simulink model "VTOLAutopilotController (minhyun-purdue's conflicted copy 2025-07-07)"  (R2024b)
settings: configuration reference "VTOLConfiguration" (kept outside this file)
undefined symbols (not defined in the file): control, controlParams, ControlSampleTime, CriticalTiltAngle, DiscIntNeverNeededParam, dspblkCoreblockFVToolHelper, flightState, FSState, FWControlParams, FWTrimSpeed, gcbh, HoverMission, R_LOOKAHEAD, ReferenceFilterDen, ReferenceFilterNum, tilt_max, tiltIni, uavParam, VTOLcontrolGains, w_trim, WindDownRate
libraries: slpidlib x32, simulink x11, uavalgslib x7, simulink_extras x1
(part 3 of 6)

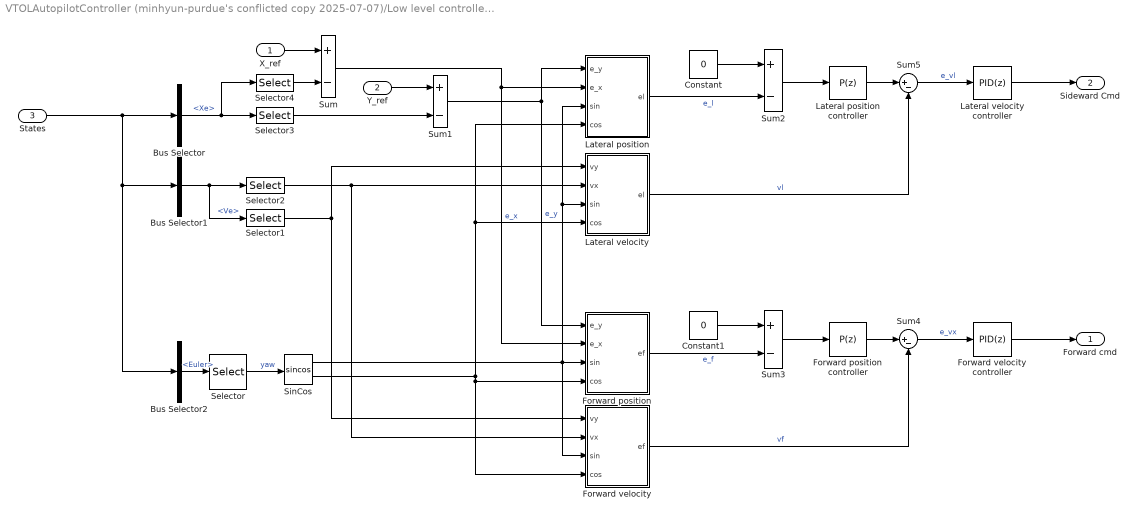
== system VTOLAutopilotController (minhyun-purdue's conflicted copy 2025-07-07)/Low level controller/Multicopter Controller/Horizontal Position Control/XY Controller ==
  X_ref : Inport
  Y_ref : Inport  Port=2
  States : Inport  Port=3
  Bus Selector : BusSelector  OutputSignals=Xe
  Bus Selector1 : BusSelector  OutputSignals=Ve
  Bus Selector2 : BusSelector  OutputSignals=Euler
  Constant : Constant  Value=0
  Constant1 : Constant  Value=0
  Forward position : Subsystem
  Forward position controller : slpidlib/PID Controller  Controller=P  Form=Parallel  TimeDomain=Discrete-time  UseExternalTs=off  SampleTime=-1  IntegratorMethod=Forward Euler  FilterMethod=Forward Euler  ControllerParametersSource=internal  P=VTOLcontrolGains.P_X  I=controlParams.I_X  UseKiTs=off  D=0.741088334151374  UseExternalDerivativeSource=off  N=1.14081860742283  UseFilter=on  TunerSelectOption=Transfer Function Based (PID Tuner App)  InitialConditionSource=internal  InitialConditionForIntegrator=0  InitialConditionForFilter=0  DifferentiatorICPrevScaledInput=0  ExternalReset=none  TrackingMode=off  Kt=1  LimitOutput=off  SatLimitsSource=internal  UpperSaturationLimit=inf  LowerSaturationLimit=-inf  LinearizeAsGain=on  AntiWindupMode=none  Kb=1  LimitIntegrator=off  UpperIntegratorSaturationLimit=inf  LowerIntegratorSaturationLimit=-inf  POutMin=[]  POutMax=[]  IOutMin=[]  IOutMax=[]  DOutMin=[]  DOutMax=[]  NOutMin=[]  NOutMax=[]  SumOutMin=[]  SumOutMax=[]  SaturationOutMin=[]  SaturationOutMax=[]  PParamMin=[]  PParamMax=[]  IParamMin=[]  IParamMax=[]  DParamMin=[]  DParamMax=[]  NParamMin=[]  NParamMax=[]  KbParamMin=[]  KbParamMax=[]  KtParamMin=[]  KtParamMax=[]  KbOutMin=[]  KbOutMax=[]  KtOutMin=[]  KtOutMax=[]  IntegratorOutMin=[]  IntegratorOutMax=[]  FilterOutMin=[]  FilterOutMax=[]  SumI1OutMin=[]  SumI1OutMax=[]  SumI2OutMin=[]  SumI2OutMax=[]  SumI3OutMin=[]  SumI3OutMax=[]  SumI4OutMin=[]  SumI4OutMax=[]  SumDOutMin=[]  SumDOutMax=[]  DifferentiatorOutMin=[]  DifferentiatorOutMax=[]  FilterDiffOutCoefMin=[]  FilterDiffOutCoefMax=[]  ReciprocalOutMin=[]  ReciprocalOutMax=[]  SumDenOutMin=[]  SumDenOutMax=[]  SumNumOutMin=[]  SumNumOutMax=[]  DivideOutMin=[]  DivideOutMax=[]  UdiffTsProdOutMin=[]  UdiffTsProdOutMax=[]  NTsProdOutMin=[]  NTsProdOutMax=[]  UintegralTsProdOutMin=[]  UintegralTsProdOutMax=[]  UngainTsProdOutMin=[]  UngainTsProdOutMax=[]  ClampingZeroOutDataTypeStr=Inherit: Inherit via back propagation  ClampingZeroOutMin=[]  ClampingZeroOutMax=[]  FilterDenConstantOutDataTypeStr=Inherit: Inherit via back propagation  FilterDenConstantOutMin=[]  FilterDenConstantOutMax=[]  PCopyOutDataTypeStr=Inherit: Inherit via back propagation  PCopyOutMin=[]  PCopyOutMax=[]  NCopyOutDataTypeStr=Inherit: Inherit via back propagation  NCopyOutMin=[]  NCopyOutMax=[]  IntegratorContinuousStateAttributes=''  IntegratorStateMustResolveToSignalObject=off  IntegratorRTWStateStorageClass=Auto  FilterContinuousStateAttributes=''  FilterStateMustResolveToSignalObject=off  FilterRTWStateStorageClass=Auto  ParallelPVariant=InternalParameters  IdealPVariant=Disabled  IVariant=Disabled  DVariant=Disabled  IntegratorVariant=Disabled  SatVariant=Disabled  AWVariant=Disabled  PCopyVariant=Disabled  TRVariant=Disabled  FdbkBlocksVariant=Forward  IdealPFdbkVariant=Disabled  SatFdbkVariant=Disabled  DerivativeFilterVariant=Disabled  NVariant=Disabled  NCopyVariant=Disabled_SignalSpec  FilterICVariant=Disabled  IntegratorICVariant=Disabled  ExternalResetVariant=Disabled  TRSumVariant=Passthrough  SumFdbkVariant=Disabled  SumVariant=Passthrough_P  TsampFilterVariant=InternalTs  TsampNgainVariant=Passthrough  TsampIntegralVariant=Disabled_SignalSpec  ExternalSaturationOutDataTypeStr=Inherit: Same as second input  DerivativeSourceVariant=Disabled  PreIntVariant=InternalPreInt
  Forward velocity : Subsystem
  Forward velocity controller : slpidlib/PID Controller  Controller=PID  Form=Parallel  TimeDomain=Discrete-time  UseExternalTs=off  SampleTime=-1  IntegratorMethod=Forward Euler  FilterMethod=Forward Euler  ControllerParametersSource=internal  P=VTOLcontrolGains.P_VX  I=VTOLcontrolGains.I_VX  UseKiTs=off  D=VTOLcontrolGains.D_VX  UseExternalDerivativeSource=off  N=VTOLcontrolGains.N_VX  UseFilter=on  TunerSelectOption=Transfer Function Based (PID Tuner App)  InitialConditionSource=internal  InitialConditionForIntegrator=0  InitialConditionForFilter=0  DifferentiatorICPrevScaledInput=0  ExternalReset=none  TrackingMode=off  Kt=1  LimitOutput=off  SatLimitsSource=internal  UpperSaturationLimit=inf  LowerSaturationLimit=-inf  LinearizeAsGain=on  AntiWindupMode=none  Kb=1  LimitIntegrator=off  UpperIntegratorSaturationLimit=inf  LowerIntegratorSaturationLimit=-inf  POutMin=[]  POutMax=[]  IOutMin=[]  IOutMax=[]  DOutMin=[]  DOutMax=[]  NOutMin=[]  NOutMax=[]  SumOutMin=[]  SumOutMax=[]  SaturationOutMin=[]  SaturationOutMax=[]  PParamMin=[]  PParamMax=[]  IParamMin=[]  IParamMax=[]  DParamMin=[]  DParamMax=[]  NParamMin=[]  NParamMax=[]  KbParamMin=[]  KbParamMax=[]  KtParamMin=[]  KtParamMax=[]  KbOutMin=[]  KbOutMax=[]  KtOutMin=[]  KtOutMax=[]  IntegratorOutMin=[]  IntegratorOutMax=[]  FilterOutMin=[]  FilterOutMax=[]  SumI1OutMin=[]  SumI1OutMax=[]  SumI2OutMin=[]  SumI2OutMax=[]  SumI3OutMin=[]  SumI3OutMax=[]  SumI4OutMin=[]  SumI4OutMax=[]  SumDOutMin=[]  SumDOutMax=[]  DifferentiatorOutMin=[]  DifferentiatorOutMax=[]  FilterDiffOutCoefMin=[]  FilterDiffOutCoefMax=[]  ReciprocalOutMin=[]  ReciprocalOutMax=[]  SumDenOutMin=[]  SumDenOutMax=[]  SumNumOutMin=[]  SumNumOutMax=[]  DivideOutMin=[]  DivideOutMax=[]  UdiffTsProdOutMin=[]  UdiffTsProdOutMax=[]  NTsProdOutMin=[]  NTsProdOutMax=[]  UintegralTsProdOutMin=[]  UintegralTsProdOutMax=[]  UngainTsProdOutMin=[]  UngainTsProdOutMax=[]  ClampingZeroOutDataTypeStr=Inherit: Inherit via back propagation  ClampingZeroOutMin=[]  ClampingZeroOutMax=[]  FilterDenConstantOutDataTypeStr=Inherit: Inherit via back propagation  FilterDenConstantOutMin=[]  FilterDenConstantOutMax=[]  PCopyOutDataTypeStr=Inherit: Inherit via back propagation  PCopyOutMin=[]  PCopyOutMax=[]  NCopyOutDataTypeStr=Inherit: Inherit via back propagation  NCopyOutMin=[]  NCopyOutMax=[]  IntegratorContinuousStateAttributes=''  IntegratorStateMustResolveToSignalObject=off  IntegratorRTWStateStorageClass=Auto  FilterContinuousStateAttributes=''  FilterStateMustResolveToSignalObject=off  FilterRTWStateStorageClass=Auto  ParallelPVariant=InternalParameters  IdealPVariant=Disabled  IVariant=InternalParameters  DVariant=InternalParameters  IntegratorVariant=Discrete  SatVariant=Disabled  AWVariant=Passthrough  PCopyVariant=Disabled  TRVariant=Disabled  FdbkBlocksVariant=Forward  IdealPFdbkVariant=Disabled  SatFdbkVariant=Disabled  DerivativeFilterVariant=ForwardEulerFilter  NVariant=InternalParameters  NCopyVariant=Disabled  FilterICVariant=InternalICsFilter  IntegratorICVariant=InternalICs  ExternalResetVariant=Disabled  TRSumVariant=Passthrough  SumFdbkVariant=Disabled  SumVariant=Sum_PID  TsampFilterVariant=InternalTs  TsampNgainVariant=Passthrough  TsampIntegralVariant=Disabled_SignalSpec  ExternalSaturationOutDataTypeStr=Inherit: Same as second input  DerivativeSourceVariant=ErrorSignal  PreIntVariant=InternalPreInt
  Lateral position : Subsystem
  Lateral position controller : slpidlib/PID Controller  Controller=P  Form=Parallel  TimeDomain=Discrete-time  UseExternalTs=off  SampleTime=-1  IntegratorMethod=Forward Euler  FilterMethod=Forward Euler  ControllerParametersSource=internal  P=VTOLcontrolGains.P_Y  I=controlParams.I_Y  UseKiTs=off  D=0.20966837124708  UseExternalDerivativeSource=off  N=1.18305565097938  UseFilter=on  TunerSelectOption=Transfer Function Based (PID Tuner App)  InitialConditionSource=internal  InitialConditionForIntegrator=0  InitialConditionForFilter=0  DifferentiatorICPrevScaledInput=0  ExternalReset=none  TrackingMode=off  Kt=1  LimitOutput=off  SatLimitsSource=internal  UpperSaturationLimit=0.4  LowerSaturationLimit=-0.4  LinearizeAsGain=on  AntiWindupMode=clamping  Kb=1  LimitIntegrator=off  UpperIntegratorSaturationLimit=inf  LowerIntegratorSaturationLimit=-inf  POutMin=[]  POutMax=[]  IOutMin=[]  IOutMax=[]  DOutMin=[]  DOutMax=[]  NOutMin=[]  NOutMax=[]  SumOutMin=[]  SumOutMax=[]  SaturationOutMin=[]  SaturationOutMax=[]  PParamMin=[]  PParamMax=[]  IParamMin=[]  IParamMax=[]  DParamMin=[]  DParamMax=[]  NParamMin=[]  NParamMax=[]  KbParamMin=[]  KbParamMax=[]  KtParamMin=[]  KtParamMax=[]  KbOutMin=[]  KbOutMax=[]  KtOutMin=[]  KtOutMax=[]  IntegratorOutMin=[]  IntegratorOutMax=[]  FilterOutMin=[]  FilterOutMax=[]  SumI1OutMin=[]  SumI1OutMax=[]  SumI2OutMin=[]  SumI2OutMax=[]  SumI3OutMin=[]  SumI3OutMax=[]  SumI4OutMin=[]  SumI4OutMax=[]  SumDOutMin=[]  SumDOutMax=[]  DifferentiatorOutMin=[]  DifferentiatorOutMax=[]  FilterDiffOutCoefMin=[]  FilterDiffOutCoefMax=[]  ReciprocalOutMin=[]  ReciprocalOutMax=[]  SumDenOutMin=[]  SumDenOutMax=[]  SumNumOutMin=[]  SumNumOutMax=[]  DivideOutMin=[]  DivideOutMax=[]  UdiffTsProdOutMin=[]  UdiffTsProdOutMax=[]  NTsProdOutMin=[]  NTsProdOutMax=[]  UintegralTsProdOutMin=[]  UintegralTsProdOutMax=[]  UngainTsProdOutMin=[]  UngainTsProdOutMax=[]  ClampingZeroOutDataTypeStr=Inherit: Inherit via back propagation  ClampingZeroOutMin=[]  ClampingZeroOutMax=[]  FilterDenConstantOutDataTypeStr=Inherit: Inherit via back propagation  FilterDenConstantOutMin=[]  FilterDenConstantOutMax=[]  PCopyOutDataTypeStr=Inherit: Inherit via back propagation  PCopyOutMin=[]  PCopyOutMax=[]  NCopyOutDataTypeStr=Inherit: Inherit via back propagation  NCopyOutMin=[]  NCopyOutMax=[]  IntegratorContinuousStateAttributes=''  IntegratorStateMustResolveToSignalObject=off  IntegratorRTWStateStorageClass=Auto  FilterContinuousStateAttributes=''  FilterStateMustResolveToSignalObject=off  FilterRTWStateStorageClass=Auto  ParallelPVariant=InternalParameters  IdealPVariant=Disabled  IVariant=Disabled  DVariant=Disabled  IntegratorVariant=Disabled  SatVariant=Disabled  AWVariant=Disabled  PCopyVariant=Disabled  TRVariant=Disabled  FdbkBlocksVariant=Forward  IdealPFdbkVariant=Disabled  SatFdbkVariant=Disabled  DerivativeFilterVariant=Disabled  NVariant=Disabled  NCopyVariant=Disabled_SignalSpec  FilterICVariant=Disabled  IntegratorICVariant=Disabled  ExternalResetVariant=Disabled  TRSumVariant=Passthrough  SumFdbkVariant=Disabled  SumVariant=Passthrough_P  TsampFilterVariant=InternalTs  TsampNgainVariant=Passthrough  TsampIntegralVariant=Disabled_SignalSpec  ExternalSaturationOutDataTypeStr=Inherit: Same as second input  DerivativeSourceVariant=Disabled  PreIntVariant=InternalPreInt
  Lateral velocity : Subsystem
  "Lateral velocity controller " : slpidlib/PID Controller  Controller=PID  Form=Parallel  TimeDomain=Discrete-time  UseExternalTs=off  SampleTime=-1  IntegratorMethod=Forward Euler  FilterMethod=Forward Euler  ControllerParametersSource=internal  P=VTOLcontrolGains.P_VY  I=VTOLcontrolGains.I_VY  UseKiTs=off  D=VTOLcontrolGains.D_VY  UseExternalDerivativeSource=off  N=VTOLcontrolGains.N_VY  UseFilter=on  TunerSelectOption=Transfer Function Based (PID Tuner App)  InitialConditionSource=internal  InitialConditionForIntegrator=0  InitialConditionForFilter=0  DifferentiatorICPrevScaledInput=0  ExternalReset=none  TrackingMode=off  Kt=1  LimitOutput=off  SatLimitsSource=internal  UpperSaturationLimit=inf  LowerSaturationLimit=-inf  LinearizeAsGain=on  AntiWindupMode=none  Kb=1  LimitIntegrator=off  UpperIntegratorSaturationLimit=inf  LowerIntegratorSaturationLimit=-inf  POutMin=[]  POutMax=[]  IOutMin=[]  IOutMax=[]  DOutMin=[]  DOutMax=[]  NOutMin=[]  NOutMax=[]  SumOutMin=[]  SumOutMax=[]  SaturationOutMin=[]  SaturationOutMax=[]  PParamMin=[]  PParamMax=[]  IParamMin=[]  IParamMax=[]  DParamMin=[]  DParamMax=[]  NParamMin=[]  NParamMax=[]  KbParamMin=[]  KbParamMax=[]  KtParamMin=[]  KtParamMax=[]  KbOutMin=[]  KbOutMax=[]  KtOutMin=[]  KtOutMax=[]  IntegratorOutMin=[]  IntegratorOutMax=[]  FilterOutMin=[]  FilterOutMax=[]  SumI1OutMin=[]  SumI1OutMax=[]  SumI2OutMin=[]  SumI2OutMax=[]  SumI3OutMin=[]  SumI3OutMax=[]  SumI4OutMin=[]  SumI4OutMax=[]  SumDOutMin=[]  SumDOutMax=[]  DifferentiatorOutMin=[]  DifferentiatorOutMax=[]  FilterDiffOutCoefMin=[]  FilterDiffOutCoefMax=[]  ReciprocalOutMin=[]  ReciprocalOutMax=[]  SumDenOutMin=[]  SumDenOutMax=[]  SumNumOutMin=[]  SumNumOutMax=[]  DivideOutMin=[]  DivideOutMax=[]  UdiffTsProdOutMin=[]  UdiffTsProdOutMax=[]  NTsProdOutMin=[]  NTsProdOutMax=[]  UintegralTsProdOutMin=[]  UintegralTsProdOutMax=[]  UngainTsProdOutMin=[]  UngainTsProdOutMax=[]  ClampingZeroOutDataTypeStr=Inherit: Inherit via back propagation  ClampingZeroOutMin=[]  ClampingZeroOutMax=[]  FilterDenConstantOutDataTypeStr=Inherit: Inherit via back propagation  FilterDenConstantOutMin=[]  FilterDenConstantOutMax=[]  PCopyOutDataTypeStr=Inherit: Inherit via back propagation  PCopyOutMin=[]  PCopyOutMax=[]  NCopyOutDataTypeStr=Inherit: Inherit via back propagation  NCopyOutMin=[]  NCopyOutMax=[]  IntegratorContinuousStateAttributes=''  IntegratorStateMustResolveToSignalObject=off  IntegratorRTWStateStorageClass=Auto  FilterContinuousStateAttributes=''  FilterStateMustResolveToSignalObject=off  FilterRTWStateStorageClass=Auto  ParallelPVariant=InternalParameters  IdealPVariant=Disabled  IVariant=InternalParameters  DVariant=InternalParameters  IntegratorVariant=Discrete  SatVariant=Disabled  AWVariant=Passthrough  PCopyVariant=Disabled  TRVariant=Disabled  FdbkBlocksVariant=Forward  IdealPFdbkVariant=Disabled  SatFdbkVariant=Disabled  DerivativeFilterVariant=ForwardEulerFilter  NVariant=InternalParameters  NCopyVariant=Disabled  FilterICVariant=InternalICsFilter  IntegratorICVariant=InternalICs  ExternalResetVariant=Disabled  TRSumVariant=Passthrough  SumFdbkVariant=Disabled  SumVariant=Sum_PID  TsampFilterVariant=InternalTs  TsampNgainVariant=Passthrough  TsampIntegralVariant=Disabled_SignalSpec  ExternalSaturationOutDataTypeStr=Inherit: Same as second input  DerivativeSourceVariant=ErrorSignal  PreIntVariant=InternalPreInt
  Selector : Selector  InputPortWidth=3  IndexOptions=Index vector (dialog)  Indices=[3]  OutputSizes=1
  Selector1 : Selector  InputPortWidth=3  IndexOptions=Index vector (dialog)  Indices=[2]  OutputSizes=1
  Selector2 : Selector  InputPortWidth=3  IndexOptions=Index vector (dialog)  Indices=[1]  OutputSizes=1
  Selector3 : Selector  InputPortWidth=3  IndexOptions=Index vector (dialog)  Indices=[2]  OutputSizes=1
  Selector4 : Selector  InputPortWidth=3  IndexOptions=Index vector (dialog)  Indices=[1]  OutputSizes=1
  SinCos : Trigonometry  Operator=sincos
  Sum{,1..3} (4 alike) : Sum  Inputs=+-
  Sum4 : Sum  Inputs=|+-
  Sum5 : Sum  Inputs=|+-
  Forward cmd : Outport
  Sideward Cmd : Outport  Port=2
  wires:
  States/1 -> Bus Selector2/1, Bus Selector1/1, Bus Selector/1
  Bus Selector/1 -> Selector4/1, Selector3/1  "<Xe>"
  Y_ref/1 -> Sum1/1
  Sum4/1 -> Forward velocity controller/1  "e_vx"
  SinCos/2 -> Forward velocity/4(cos), Forward position/4(cos), Lateral position/4(cos), Lateral velocity/4(cos)
  Selector/1 -> SinCos/1  "yaw"
  Lateral position/1(el) -> Sum2/2  "e_l"
  Sum1/1 -> Lateral position/1(e_y), Forward position/1(e_y)  "e_y"
  SinCos/1 -> Lateral velocity/3(sin), Lateral position/3(sin), Forward position/3(sin), Forward velocity/3(sin)
  Lateral velocity/1(el) -> Sum5/2  "vl"
  Forward position/1(ef) -> Sum3/2  "e_f"
  Forward velocity/1(ef) -> Sum4/2  "vf"
  Lateral position controller/1 -> Sum5/1
  Forward position controller/1 -> Sum4/1
  Sum5/1 -> "Lateral velocity controller "/1  "e_vl"
  "Lateral velocity controller "/1 -> Sideward Cmd/1
  Forward velocity controller/1 -> Forward cmd/1
  Constant/1 -> Sum2/1
  Sum2/1 -> Lateral position controller/1
  Constant1/1 -> Sum3/1
  Sum3/1 -> Forward position controller/1
  Bus Selector2/1 -> Selector/1  "<Euler>"
  Selector2/1 -> Forward velocity/2(vx), Lateral velocity/2(vx)
  Selector1/1 -> Lateral velocity/1(vy), Forward velocity/1(vy)
  Bus Selector1/1 -> Selector2/1, Selector1/1  "<Ve>"
  Selector3/1 -> Sum1/2
  Selector4/1 -> Sum/2
  Sum/1 -> Forward position/2(e_x), Lateral position/2(e_x)  "e_x"
  X_ref/1 -> Sum/1

== system VTOLAutopilotController (minhyun-purdue's conflicted copy 2025-07-07)/Low level controller/Multicopter Controller/Subsystem/Triggered Subsystem ==
  YawHold : Inport
  Trigger : TriggerPort  VariantControl=(inherit)
  Reference : Outport
  wires:
  YawHold/1 -> Reference/1

== system VTOLAutopilotController (minhyun-purdue's conflicted copy 2025-07-07)/Low level controller/Scheduler/FixedWingScheduler/Switch Case Action Subsystem ==
  note: No control allocated from fixed wing during hover.
  Action Port : ActionPort  ActionPortLabel=case [ Hover ]:
  Bus Creator : BusCreator  Inputs=4
  Constant{,1..3} (4 alike) : Constant  Value=0
  FixedWingControls : Outport  OutDataTypeStr=Bus: FixedWingCtrlBus
  wires:
  Bus Creator/1 -> FixedWingControls/1
  Constant/1 -> Bus Creator/1  "dA"
  Constant1/1 -> Bus Creator/2  "dE"
  Constant2/1 -> Bus Creator/3  "dR"
  Constant3/1 -> Bus Creator/4  "dT"

== system VTOLAutopilotController (minhyun-purdue's conflicted copy 2025-07-07)/Low level controller/Scheduler/FixedWingScheduler/Switch Case Action Subsystem1 ==
  FixedWingActuators : Inport  OutDataTypeStr=Bus: FixedWingCtrlBus
  TransitionDone : Inport  Port=2
  Action Port : ActionPort  ActionPortLabel=case [ Transition ]:
  Bus Creator : BusCreator  Inputs=4  OutDataTypeStr=Bus: FixedWingCtrlBus
  Constant : Constant  Value=0
  Constant1 : Constant  Value=controlParams.FWElevatorTrim
  Constant2 : Constant  Value=0
  Constant3 : Constant  Value=0
  Switch : Switch  Criteria=u2 > Threshold  SaturateOnIntegerOverflow=off  InputSameDT=off
  FixedWingControls : Outport  OutDataTypeStr=Bus: FixedWingCtrlBus
  wires:
  Bus Creator/1 -> Switch/3
  Constant/1 -> Bus Creator/1  "dA"
  Constant1/1 -> Bus Creator/2  "dE"
  Constant2/1 -> Bus Creator/3  "dR"
  Constant3/1 -> Bus Creator/4  "dT"
  FixedWingActuators/1 -> Switch/1
  Switch/1 -> FixedWingControls/1
  TransitionDone/1 -> Switch/2

== system VTOLAutopilotController (minhyun-purdue's conflicted copy 2025-07-07)/Low level controller/Scheduler/FixedWingScheduler/Switch Case Action Subsystem2 ==
  FixedWingActuators : Inport  OutDataTypeStr=Bus: FixedWingCtrlBus
  Action Port : ActionPort  ActionPortLabel=case [ FixedWing ]:
  FixedWingControls : Outport  OutDataTypeStr=Bus: FixedWingCtrlBus
  wires:
  FixedWingActuators/1 -> FixedWingControls/1

== system VTOLAutopilotController (minhyun-purdue's conflicted copy 2025-07-07)/Low level controller/Scheduler/FixedWingScheduler/Switch Case Action Subsystem3 ==
  note: No control allocated from fixed wing during hover.
  Action Port : ActionPort  ActionPortLabel=case [ BackTransition ]:
  Bus Creator : BusCreator  Inputs=4
  Constant{,1..3} (4 alike) : Constant  Value=0
  FixedWingControls : Outport  OutDataTypeStr=Bus: FixedWingCtrlBus
  wires:
  Bus Creator/1 -> FixedWingControls/1
  Constant/1 -> Bus Creator/1  "dA"
  Constant1/1 -> Bus Creator/2  "dE"
  Constant3/1 -> Bus Creator/4  "dT"
  Constant2/1 -> Bus Creator/3  "dR"

== system VTOLAutopilotController (minhyun-purdue's conflicted copy 2025-07-07)/Low level controller/Scheduler/Subsystem/Actuator To Voltage ==
  note: #2, 25/05/20, MH, Fixed
      | The rotor rotational speed command should be
      | normalized to [rad/s].Previously, division by 2PI
      | was omitted in the command block,
      | while the 'Rotor Assembly' block multiplies
      | the input by 2PI, leading to increased gains.
  Motor Commands : Inport
  Bus Creator : BusCreator  Inputs=6  OutDataTypeStr=Bus: RotorCtrlBus
  Bus Selector : BusSelector  OutputSignals=w1,w2,w3,w4,Tilt1,Tilt2
  Gain{,1..2,4} (4 alike) : Gain  Gain=1/(uavParam.motor.RPMMAX/60)
  Gain3 : Gain  Gain=1/(pi/2)
  Gain5 : Gain  Gain=1/(pi/2)
  Gain{6..9} (4 alike) : Gain  Gain=1/(2*pi)
  Saturation{,1..3} (4 alike) : Saturate  UpperLimit=controlParams.maxPWM  LowerLimit=controlParams.minPWM
  Saturation4 : Saturate  UpperLimit=1  LowerLimit=0
  Saturation5 : Saturate  UpperLimit=1  LowerLimit=0
  To PWM : Outport
  wires:
  Motor Commands/1 -> Bus Selector/1
  Bus Selector/1 -> Gain/1  "<w1>"
  Bus Selector/3 -> Gain1/1  "<w3>"
  Bus Selector/2 -> Gain4/1  "<w2>"
  Bus Selector/4 -> Gain2/1  "<w4>"
  Bus Selector/5 -> Gain3/1  "<Tilt1>"
  Bus Selector/6 -> Gain5/1  "<Tilt2>"
  Gain/1 -> Gain6/1  "w1"
  Gain4/1 -> Gain7/1  "w2"
  Gain1/1 -> Gain8/1  "w3"
  Gain2/1 -> Gain9/1  "w4"
  Gain3/1 -> Saturation4/1
  Gain5/1 -> Saturation5/1
  Bus Creator/1 -> To PWM/1
  Gain6/1 -> Saturation/1
  Gain7/1 -> Saturation1/1
  Gain8/1 -> Saturation2/1
  Gain9/1 -> Saturation3/1
  Saturation/1 -> Bus Creator/1  "w1"
  Saturation1/1 -> Bus Creator/2  "w2"
  Saturation2/1 -> Bus Creator/3  "w3"
  Saturation3/1 -> Bus Creator/4  "w4"
  Saturation4/1 -> Bus Creator/5  "Tilt1"
  Saturation5/1 -> Bus Creator/6  "Tilt2"

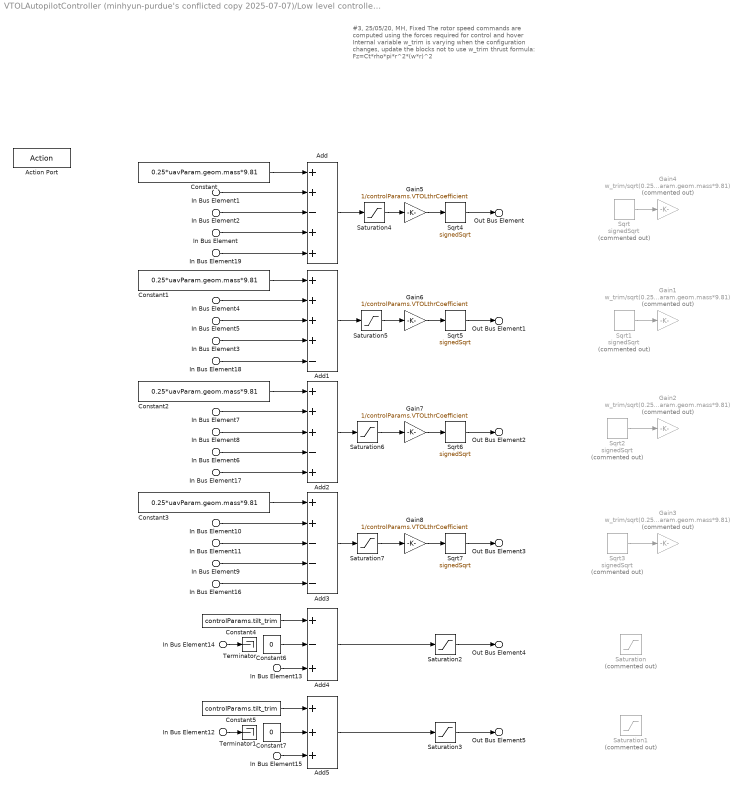
== system VTOLAutopilotController (minhyun-purdue's conflicted copy 2025-07-07)/Low level controller/Scheduler/Subsystem/Switch Case Action Subsystem ==
  note: #3, 25/05/20, MH, Fixed
      | The rotor speed commands are computed using
      | the forces required for control and hover
      | Internal variable w_trim is varying when the
      | configuration changes, update the blocks not to
      | use w_trim
      | thrust formula: Fz=Ct*rho*pi*r^2*(w*r)^2
  In Bus Element{,3,6,9} (4 alike) : Inport  PortName=MixerCommands  Element=w_theta
  In Bus Element{1,4,7,10} (4 alike) : Inport  PortName=MixerCommands  Element=w_z
  In Bus Element{2,5,8,11} (4 alike) : Inport  PortName=MixerCommands  Element=w_phi
  In Bus Element13 : Inport  PortName=MixerCommands  Element=l_x
  In Bus Element15 : Inport  PortName=MixerCommands  Element=l_x
  In Bus Element{12,14,16..19} (6 alike) : Inport  PortName=MixerCommands  Element=w_psi
  Action Port : ActionPort  ActionPortLabel=case [ Hover ]:
  Add : Sum  Inputs=++-++
  Add1 : Sum  Inputs=++++-
  Add2 : Sum  Inputs=+++-+
  Add3 : Sum  Inputs=++---
  Add4 : Sum  Inputs=+-+
  Add5 : Sum  Inputs=+++
  Constant{,1..3} (4 alike) : Constant  Value=0.25*uavParam.geom.mass*9.81
  Constant4 : Constant  Value=controlParams.tilt_trim
  Constant5 : Constant  Value=controlParams.tilt_trim
  Constant6 : Constant  Value=0
  Constant7 : Constant  Value=0
  Gain{1..4} (4 alike) : Gain  Commented=on  Gain=w_trim/sqrt(0.25*uavParam.geom.mass*9.81)
  Gain{5..8} (4 alike) : Gain  Gain=1/controlParams.VTOLthrCoefficient
  Saturation : Saturate  Commented=on  UpperLimit=tilt_max  LowerLimit=-tilt_max
  Saturation1 : Saturate  Commented=on  UpperLimit=tilt_max  LowerLimit=-tilt_max
  Saturation2 : Saturate  UpperLimit=tilt_max  LowerLimit=-tilt_max
  Saturation3 : Saturate  UpperLimit=tilt_max  LowerLimit=-tilt_max
  Saturation{4..7} (4 alike) : Saturate  UpperLimit=inf  LowerLimit=0
  Sqrt{,1..3} (4 alike) : Sqrt  Commented=on  Operator=signedSqrt
  Sqrt{4..7} (4 alike) : Sqrt  Operator=signedSqrt
  Terminator : Terminator
  Terminator1 : Terminator
  Out Bus Element : Outport  PortName=Actuator  Element=w1
  Out Bus Element1 : Outport  PortName=Actuator  Element=w2
  Out Bus Element2 : Outport  PortName=Actuator  Element=w3
  Out Bus Element3 : Outport  PortName=Actuator  Element=w4
  Out Bus Element4 : Outport  PortName=Actuator  Element=Tilt1
  Out Bus Element5 : Outport  PortName=Actuator  Element=Tilt2
  wires:
  Constant5/1 -> Add5/1
  Constant2/1 -> Add2/1
  Constant1/1 -> Add1/1
  Constant4/1 -> Add4/1
  Constant/1 -> Add/1
  Constant3/1 -> Add3/1
  Add/1 -> Saturation4/1
  Add1/1 -> Saturation5/1
  Add2/1 -> Saturation6/1
  Add3/1 -> Saturation7/1
  In Bus Element13/1 -> Add4/3
  In Bus Element15/1 -> Add5/3
  Saturation2/1 -> Out Bus Element4/1
  Add4/1 -> Saturation2/1
  Add5/1 -> Saturation3/1
  Saturation3/1 -> Out Bus Element5/1
  Saturation4/1 -> Gain5/1
  Saturation5/1 -> Gain6/1
  Saturation6/1 -> Gain7/1
  Saturation7/1 -> Gain8/1
  Sqrt4/1 -> Out Bus Element/1
  Sqrt5/1 -> Out Bus Element1/1
  Sqrt6/1 -> Out Bus Element2/1
  Sqrt7/1 -> Out Bus Element3/1
  In Bus Element2/1 -> Add/3
  In Bus Element/1 -> Add/4
  In Bus Element5/1 -> Add1/3
  In Bus Element3/1 -> Add1/4
  In Bus Element8/1 -> Add2/3
  In Bus Element11/1 -> Add3/3
  In Bus Element9/1 -> Add3/4
  In Bus Element6/1 -> Add2/4
  Sqrt/1 -> Gain4/1
  Sqrt3/1 -> Gain3/1
  Sqrt2/1 -> Gain2/1
  Sqrt1/1 -> Gain1/1
  Gain5/1 -> Sqrt4/1
  Gain6/1 -> Sqrt5/1
  Gain7/1 -> Sqrt6/1
  Gain8/1 -> Sqrt7/1
  In Bus Element1/1 -> Add/2
  In Bus Element4/1 -> Add1/2
  In Bus Element7/1 -> Add2/2
  In Bus Element10/1 -> Add3/2
  In Bus Element19/1 -> Add/5
  In Bus Element16/1 -> Add3/5
  In Bus Element17/1 -> Add2/5
  In Bus Element18/1 -> Add1/5
  In Bus Element14/1 -> Terminator/1
  In Bus Element12/1 -> Terminator1/1
  Constant6/1 -> Add4/2
  Constant7/1 -> Add5/2

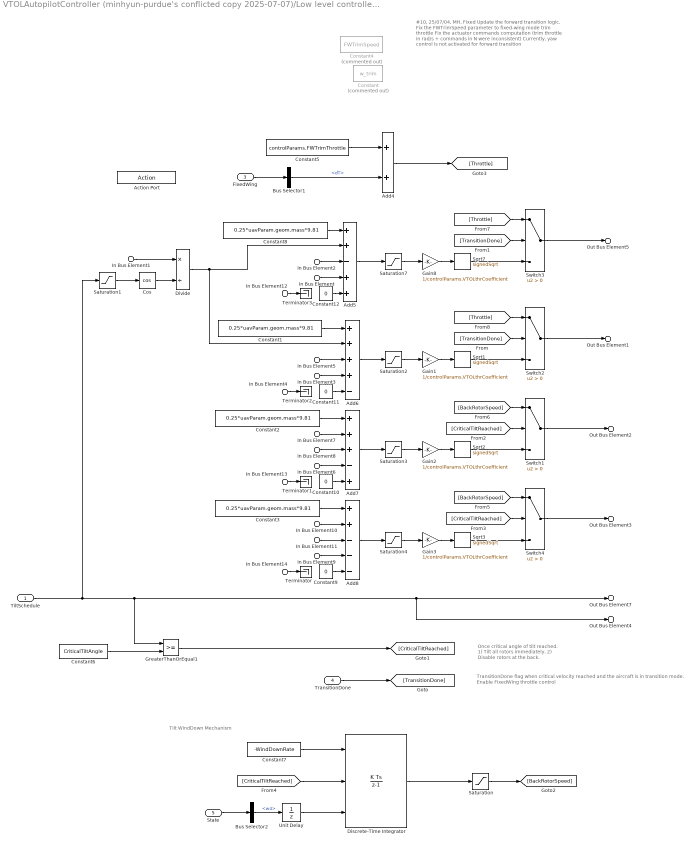
== system VTOLAutopilotController (minhyun-purdue's conflicted copy 2025-07-07)/Low level controller/Scheduler/Subsystem/Switch Case Action Subsystem1 ==
  note: Tilt WindDown Mechanism
  note: Once critical angle of tilt reached.
      | 1) Tilt all rotors immediately.
      | 2) Disable rotors at the back.
  note: TransitionDone flag when critical velocity reached and the aircraft is in transition mode.
      | Enable FixedWing throttle control
  note: #10, 25/07/04, MH, Fixed
      | Update the forward transition logic.
      | Fix the FWTrimSpeed parameter to fixed-wing
      | mode trim throttle
      | Fix the actuator commands computation
      | (trim throttle in rad/s + commands in N were
      | inconsistent)
      | Currently, yaw control is not activated for
      | forward transition
  TiltSchedule : Inport
  In Bus Element{,3,6,9} (4 alike) : Inport  Port=2  PortName=MixerCommands  Element=w_theta
  In Bus Element1 : Inport  Port=2  PortName=MixerCommands  Element=w_z
  In Bus Element7 : Inport  Port=2  PortName=MixerCommands  Element=w_z
  In Bus Element10 : Inport  Port=2  PortName=MixerCommands  Element=w_z
  In Bus Element{2,5,8,11} (4 alike) : Inport  Port=2  PortName=MixerCommands  Element=w_phi
  In Bus Element{4,12..14} (4 alike) : Inport  Port=2  PortName=MixerCommands  Element=w_psi
  FixedWing : Inport  Port=3
  TransitionDone : Inport  Port=4
  State : Inport  Port=5
  Action Port : ActionPort  ActionPortLabel=case [ Transition ]:
  Add4 : Sum
  Add5 : Sum  Inputs=++-++
  Add6 : Sum  Inputs=++++-
  Add7 : Sum  Inputs=+++-+
  Add8 : Sum  Inputs=++---
  Bus Selector1 : BusSelector  OutputSignals=dT
  Bus Selector2 : BusSelector  OutputSignals=RotorParameters.w4
  Constant : Constant  Commented=on  Value=w_trim
  Constant{1..3,8} (4 alike) : Constant  Value=0.25*uavParam.geom.mass*9.81
  Constant{9..12} (4 alike) : Constant  Value=0
  Constant4 : Constant  Commented=on  Value=FWTrimSpeed
  Constant5 : Constant  Value=controlParams.FWTrimThrottle
  Constant6 : Constant  Value=CriticalTiltAngle
  Constant7 : Constant  Value=-WindDownRate
  Cos : Trigonometry  Operator=cos
  Discrete-Time Integrator : DiscreteIntegrator  ExternalReset=either  InitialConditionSource=external  SampleTime=0.005  ICPrevOutput=DiscIntNeverNeededParam  ICPrevScaledInput=DiscIntNeverNeededParam
  Divide : Product  Inputs=*/
  Gain{1..3,8} (4 alike) : Gain  Gain=1/controlParams.VTOLthrCoefficient
  GreaterThanOrEqual1 : RelationalOperator  OutDataTypeStr=boolean  RndMeth=Simplest  InputSameDT=off
  Saturation : Saturate  UpperLimit=Inf  LowerLimit=0
  Saturation1 : Saturate  UpperLimit=CriticalTiltAngle  LowerLimit=-CriticalTiltAngle
  Saturation{2..4,7} (4 alike) : Saturate  UpperLimit=inf  LowerLimit=0
  Sqrt{1..3,7} (4 alike) : Sqrt  Operator=signedSqrt
  Switch{1..4} (4 alike) : Switch  Criteria=u2 > Threshold  SaturateOnIntegerOverflow=off  InputSameDT=off
  Terminator{,1..3} (4 alike) : Terminator
  Unit Delay : UnitDelay  SampleTime=-1  HasFrameUpgradeWarning=on
  Out Bus Element5 : Outport  PortName=Actuator  Element=w1
  Out Bus Element1 : Outport  PortName=Actuator  Element=w2
  Out Bus Element2 : Outport  PortName=Actuator  Element=w3
  Out Bus Element3 : Outport  PortName=Actuator  Element=w4
  Out Bus Element7 : Outport  PortName=Actuator  Element=Tilt1
  Out Bus Element4 : Outport  PortName=Actuator  Element=Tilt2
  wires:
  TiltSchedule/1 -> GreaterThanOrEqual1/1, Out Bus Element4/1, Out Bus Element7/1, Saturation1/1
  In Bus Element9/1 -> Add8/4
  In Bus Element6/1 -> Add7/4
  In Bus Element8/1 -> Add7/3
  Constant3/1 -> Add8/1
  In Bus Element/1 -> Add5/4
  In Bus Element10/1 -> Add8/2
  Constant1/1 -> Add6/1
  In Bus Element11/1 -> Add8/3
  In Bus Element3/1 -> Add6/4
  In Bus Element2/1 -> Add5/3
  In Bus Element7/1 -> Add7/2
  Constant2/1 -> Add7/1
  In Bus Element5/1 -> Add6/3
  FixedWing/1 -> Bus Selector1/1
  Bus Selector1/1 -> Add4/2  "<dT>"
  [TransitionDone] -> Switch3/2
  Constant6/1 -> GreaterThanOrEqual1/2
  GreaterThanOrEqual1/1 -> [CriticalTiltReached]
  [CriticalTiltReached] -> Switch1/2
  [BackRotorSpeed] -> Switch1/1
  [CriticalTiltReached] -> Switch4/2
  [BackRotorSpeed] -> Switch4/1
  TransitionDone/1 -> [TransitionDone]
  Bus Selector2/1 -> Unit Delay/1  "<w4>"
  Constant7/1 -> Discrete-Time Integrator/1
  [CriticalTiltReached] -> Discrete-Time Integrator/2
  Discrete-Time Integrator/1 -> Saturation/1
  Saturation/1 -> [BackRotorSpeed]
  State/1 -> Bus Selector2/1
  Unit Delay/1 -> Discrete-Time Integrator/3
  Add4/1 -> [Throttle]
  [Throttle] -> Switch3/1
  Cos/1 -> Divide/2
  Saturation1/1 -> Cos/1
  In Bus Element1/1 -> Divide/1
  Divide/1 -> Add5/2, Add6/2
  Switch3/1 -> Out Bus Element5/1
  Switch1/1 -> Out Bus Element2/1
  Switch4/1 -> Out Bus Element3/1
  Constant5/1 -> Add4/1
  Gain8/1 -> Sqrt7/1
  Saturation7/1 -> Gain8/1
  Constant8/1 -> Add5/1
  Add5/1 -> Saturation7/1
  Sqrt7/1 -> Switch3/3
  [TransitionDone] -> Switch2/2
  [Throttle] -> Switch2/1
  Switch2/1 -> Out Bus Element1/1
  Saturation2/1 -> Gain1/1
  Gain1/1 -> Sqrt1/1
  Add6/1 -> Saturation2/1
  Sqrt1/1 -> Switch2/3
  Gain2/1 -> Sqrt2/1
  Saturation3/1 -> Gain2/1
  Add7/1 -> Saturation3/1
  Sqrt2/1 -> Switch1/3
  Gain3/1 -> Sqrt3/1
  Saturation4/1 -> Gain3/1
  Add8/1 -> Saturation4/1
  Sqrt3/1 -> Switch4/3
  Constant9/1 -> Add8/5
  In Bus Element14/1 -> Terminator/1
  Constant10/1 -> Add7/5
  In Bus Element13/1 -> Terminator1/1
  Constant11/1 -> Add6/5
  In Bus Element4/1 -> Terminator2/1
  Constant12/1 -> Add5/5
  In Bus Element12/1 -> Terminator3/1

== system VTOLAutopilotController (minhyun-purdue's conflicted copy 2025-07-07)/Low level controller/Scheduler/Subsystem/Switch Case Action Subsystem2 ==
  note: Tilt WindDown Mechanism
  In Bus Element2 : Inport  PortName=FixedWingCtrlBus  Element=dT
  In Bus Element1 : Inport  PortName=FixedWingCtrlBus  Element=dT
  TransitionDone : Inport  Port=2
  State : Inport  Port=3
  Action Port : ActionPort  ActionPortLabel=case [ FixedWing ]:
  Add : Sum
  Add1 : Sum
  Bus Selector2 : BusSelector  OutputSignals=RotorParameters.w4
  Constant : Constant  Commented=on  Value=FWTrimSpeed
  Constant1 : Constant  Value=-WindDownRate
  Constant4 : Constant  Value=pi/2
  Constant5 : Constant  Value=controlParams.FWTrimThrottle
  Constant7 : Constant  Value=pi/2
  Discrete-Time Integrator : DiscreteIntegrator  ExternalReset=rising  InitialConditionSource=external  SampleTime=0.005  ICPrevOutput=DiscIntNeverNeededParam  ICPrevScaledInput=DiscIntNeverNeededParam
  Saturation : Saturate  UpperLimit=Inf  LowerLimit=0
  Saturation1 : Saturate  UpperLimit=Inf  LowerLimit=0
  Saturation2 : Saturate  UpperLimit=Inf  LowerLimit=0
  Out Bus Element : Outport  PortName=Actuator  Element=w1
  Out Bus Element1 : Outport  PortName=Actuator  Element=w2
  Out Bus Element2 : Outport  PortName=Actuator  Element=w3
  Out Bus Element3 : Outport  PortName=Actuator  Element=w4
  Out Bus Element7 : Outport  PortName=Actuator  Element=Tilt1
  Out Bus Element4 : Outport  PortName=Actuator  Element=Tilt2
  wires:
  Add1/1 -> Saturation1/1
  Constant4/1 -> Out Bus Element4/1
  [BackRotorSpeed] -> Out Bus Element2/1
  Constant7/1 -> Out Bus Element7/1
  In Bus Element2/1 -> Add1/2
  Add/1 -> Saturation/1
  In Bus Element1/1 -> Add/2
  Saturation/1 -> Out Bus Element/1
  Saturation1/1 -> Out Bus Element1/1
  [BackRotorSpeed] -> Out Bus Element3/1
  Bus Selector2/1 -> Discrete-Time Integrator/3  "<w4>"
  Saturation2/1 -> [BackRotorSpeed]
  State/1 -> Bus Selector2/1
  Constant1/1 -> Discrete-Time Integrator/1
  Discrete-Time Integrator/1 -> Saturation2/1
  TransitionDone/1 -> Discrete-Time Integrator/2
  Constant5/1 -> Add/1, Add1/1

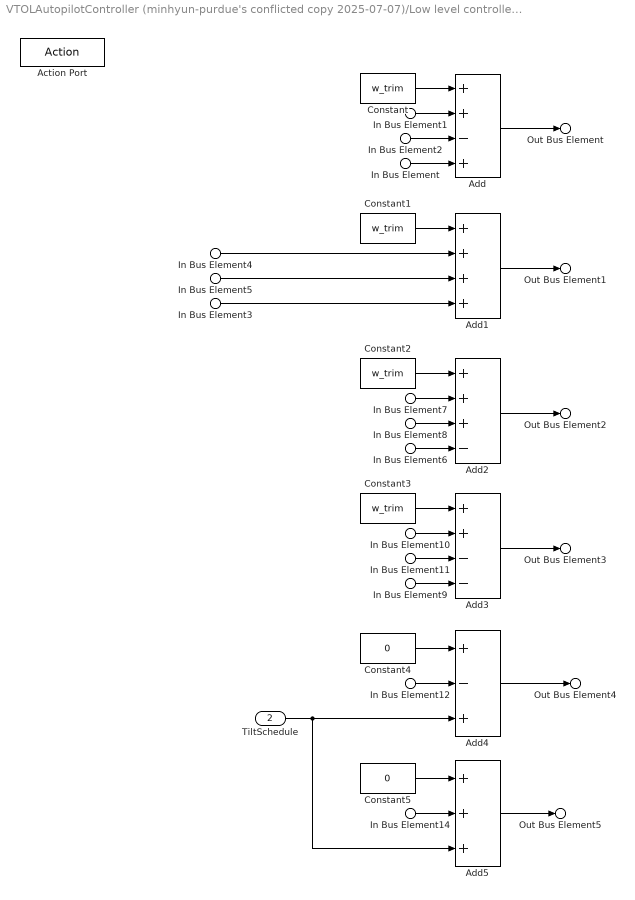
== system VTOLAutopilotController (minhyun-purdue's conflicted copy 2025-07-07)/Low level controller/Scheduler/Subsystem/Switch Case Action Subsystem3 ==
  In Bus Element{,3,6,9} (4 alike) : Inport  PortName=MixerCommands  Element=w_theta
  In Bus Element{1,4,7,10} (4 alike) : Inport  PortName=MixerCommands  Element=w_z
  In Bus Element{2,5,8,11} (4 alike) : Inport  PortName=MixerCommands  Element=w_phi
  In Bus Element12 : Inport  PortName=MixerCommands  Element=w_psi
  In Bus Element14 : Inport  PortName=MixerCommands  Element=w_psi
  TiltSchedule : Inport  Port=2
  Action Port : ActionPort  ActionPortLabel=case [ BackTransition ]:
  Add : Sum  Inputs=++-+
  Add1 : Sum  Inputs=++++
  Add2 : Sum  Inputs=+++-
  Add3 : Sum  Inputs=++--
  Add4 : Sum  Inputs=+-+
  Add5 : Sum  Inputs=+++
  Constant{,1..3} (4 alike) : Constant  Value=w_trim
  Constant4 : Constant  Value=0
  Constant5 : Constant  Value=0
  Out Bus Element : Outport  PortName=Actuator  Element=w1
  Out Bus Element1 : Outport  PortName=Actuator  Element=w2
  Out Bus Element2 : Outport  PortName=Actuator  Element=w3
  Out Bus Element3 : Outport  PortName=Actuator  Element=w4
  Out Bus Element4 : Outport  PortName=Actuator  Element=Tilt1
  Out Bus Element5 : Outport  PortName=Actuator  Element=Tilt2
  wires:
  In Bus Element4/1 -> Add1/2
  In Bus Element2/1 -> Add/3
  In Bus Element5/1 -> Add1/3
  In Bus Element3/1 -> Add1/4
  In Bus Element/1 -> Add/4
  In Bus Element11/1 -> Add3/3
  In Bus Element8/1 -> Add2/3
  Constant2/1 -> Add2/1
  In Bus Element9/1 -> Add3/4
  In Bus Element6/1 -> Add2/4
  Constant1/1 -> Add1/1
  In Bus Element10/1 -> Add3/2
  In Bus Element1/1 -> Add/2
  Add1/1 -> Out Bus Element1/1
  Constant/1 -> Add/1
  Constant3/1 -> Add3/1
  Add/1 -> Out Bus Element/1
  Add2/1 -> Out Bus Element2/1
  Add3/1 -> Out Bus Element3/1
  In Bus Element7/1 -> Add2/2
  Constant4/1 -> Add4/1
  In Bus Element12/1 -> Add4/2
  TiltSchedule/1 -> Add5/3, Add4/3
  Constant5/1 -> Add5/1
  In Bus Element14/1 -> Add5/2
  Add4/1 -> Out Bus Element4/1
  Add5/1 -> Out Bus Element5/1

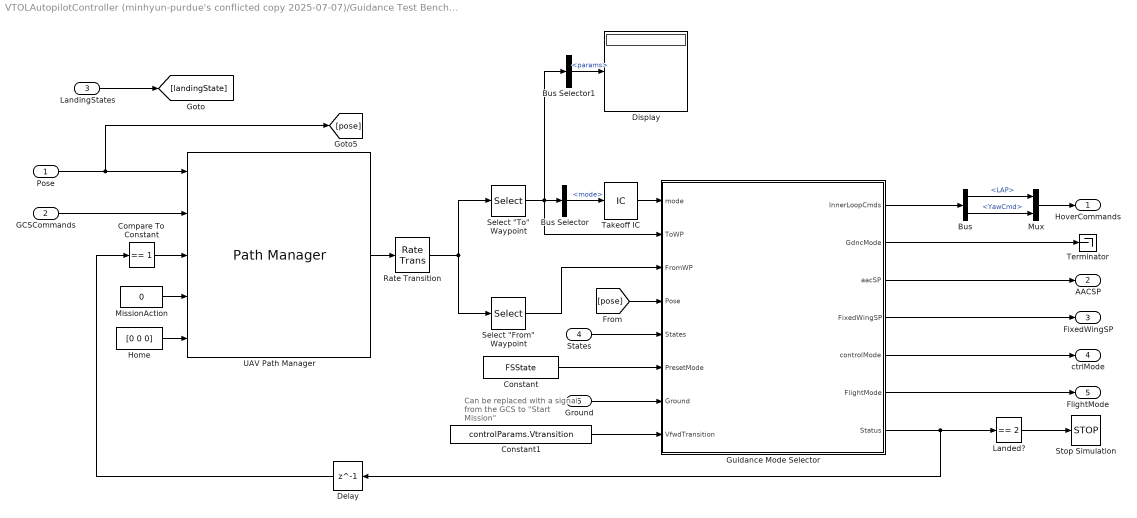
== system VTOLAutopilotController (minhyun-purdue's conflicted copy 2025-07-07)/Guidance Test Bench/ControlType/Guidance Testbench/Guidance Logic/Guidance Stateflow ==
  note: Can be replaced with a signal from the GCS to "Start Mission"
  Pose : Inport
  GCSCommands : Inport  Port=2
  LandingStates : Inport  Port=3
  States : Inport  Port=4
  Ground : Inport  Port=5
  "Bus " : BusSelector  OutputSignals=LAP,YawCmd
  Bus Selector : BusSelector  OutputSignals=mode
  Bus Selector1 : BusSelector  OutputSignals=params
  Compare To Constant : simulink/Logic and Bit Operations/Compare To Constant  relop===  const=1  OutDataTypeStr=boolean
  Constant : Constant  Value=FSState
  Constant1 : Constant  Value=controlParams.Vtransition
  Delay : Delay  DelayLength=1  InitialCondition=0
  Display : Display
  Guidance Mode Selector : Stateflow chart  TreatAsAtomicUnit=on  SystemSampleTime=0.02
      settings: PortSchema="{\"entries\":[{\"content\":{\"sides\":[{\"content\":{\"connectorIds\":[\"In1\",\"In2\",\"In3\",\"In4\",\"In5\",\"In6\",\"In7\",\"In8\"]},\"type\":\"ConnectorPlacement.EquallySpacedRectSide\",\"uuid\":\"a9cfd0e2-196c-422d-b359-9161a47768c9\"},{\"content\":{\"connectorIds\":[\"Out7\",\"Out2\",\"Out3\",\"Out4\",\"Out5\",\"Out6\",\"Out1\"],\"side\":\"RIGHT\"},\"type\":\"ConnectorPlacement.EquallySpacedRectSide\",\"uuid\":\"4fed41ae-e7cf-4de3-8bdb-9e24e7d8b079\"},{\"content\":{\"side\":\"TOP\"},\"type\":\"ConnectorPlacement.EquallySpacedRectSide\",\"uuid\":\"2d49ff20-2f63-498d-ac9d-820eae01f794\"}]},\"type\":\"ConnectorPlacement.EquallySpacedConnector\",\"uuid\":\"88d403f4-ad96-40f9-9697-84906f26a8bf\"}],\"packageUris\":[\"http://schema.mathworks.com/mf0/Connector/R2020b\"],\"version\":\"1.0\"}"
  Home : Constant  Value=[0 0 0]  OutDataTypeStr=double
  Landed? : simulink/Logic and Bit Operations/Compare To Constant  relop===  const=2  OutDataTypeStr=boolean
  MissionAction : Constant  Value=0  OutDataTypeStr=uint8
  Mux : Mux  Inputs=2
  Rate Transition : RateTransition
  "Select \"From\" Waypoint" : Selector  InputPortWidth=2  IndexOptions=Index vector (dialog)  Indices=2  OutputSizes=1
  "Select \"To\" Waypoint" : Selector  InputPortWidth=2  IndexOptions=Index vector (dialog)  Indices=1  OutputSizes=1
  Stop Simulation : Stop
  Takeoff IC : InitialCondition
  Terminator : Terminator
  UAV Path Manager : uavalgslib/Path Manager  UAVType=multirotor  LoiterRadius=25  dataType=double  inputBusName='doubleUavPathManager'  SimulateUsing=Code generation
  HoverCommands : Outport
  AACSP : Outport  Port=2
  FixedWingSP : Outport  Port=3
  ctrlMode : Outport  Port=4
  FlightMode : Outport  Port=5
  wires:
  Takeoff IC/1 -> Guidance Mode Selector/1(mode)
  MissionAction/1 -> UAV Path Manager/4
  Guidance Mode Selector/1(Status) -> Delay/1, Landed?/1
  Home/1 -> UAV Path Manager/5
  GCSCommands/1 -> UAV Path Manager/2
  UAV Path Manager/1 -> Rate Transition/1
  Bus Selector/1 -> Takeoff IC/1  "<mode>"
  [pose] -> Guidance Mode Selector/4(Pose)
  Compare To Constant/1 -> UAV Path Manager/3
  "Select \"To\" Waypoint"/1 -> Bus Selector1/1, Guidance Mode Selector/2(ToWP), Bus Selector/1
  "Select \"From\" Waypoint"/1 -> Guidance Mode Selector/3(FromWP)
  Landed?/1 -> Stop Simulation/1
  Guidance Mode Selector/2(GdncMode) -> Terminator/1
  Delay/1 -> Compare To Constant/1
  LandingStates/1 -> [landingState]
  States/1 -> Guidance Mode Selector/5(States)
  Guidance Mode Selector/5(controlMode) -> ctrlMode/1
  Guidance Mode Selector/3(aacSP) -> AACSP/1
  Guidance Mode Selector/4(FixedWingSP) -> FixedWingSP/1
  Guidance Mode Selector/6(FlightMode) -> FlightMode/1
  Constant/1 -> Guidance Mode Selector/6(PresetMode)
  "Bus "/1 -> Mux/1  "<LAP>"
  "Bus "/2 -> Mux/2  "<YawCmd>"
  Mux/1 -> HoverCommands/1
  Guidance Mode Selector/7(InnerLoopCmds) -> "Bus "/1
  Ground/1 -> Guidance Mode Selector/7(Ground)
  Pose/1 -> UAV Path Manager/1, [pose]
  Rate Transition/1 -> "Select \"From\" Waypoint"/1, "Select \"To\" Waypoint"/1
  Constant1/1 -> Guidance Mode Selector/8(VfwdTransition)
  Bus Selector1/1 -> Display/1  "<params>"

== system VTOLAutopilotController (minhyun-purdue's conflicted copy 2025-07-07)/Guidance Test Bench/ControlType/Guidance Testbench/Guidance Logic/Interface ==
  UAVState : Inport
  Bus Creator : BusCreator  Inputs=5
  Bus Selector : BusSelector  OutputSignals=Xe,Ve
  Demux : Demux  Outputs=3
  Selector : Selector  InputPortWidth=3  IndexOptions=Index vector (dialog)  Indices=[1]  OutputSizes=1
  Selector1 : Selector  InputPortWidth=3  IndexOptions=Index vector (dialog)  Indices=[2]  OutputSizes=1
  States : Outport
  wires:
  Demux/2 -> Bus Creator/2  "y"
  UAVState/1 -> Bus Selector/1
  Bus Selector/2 -> Selector/1, Selector1/1  "<Ve>"
  Bus Selector/1 -> Demux/1  "<Xe>"
  Demux/1 -> Bus Creator/1  "x"
  Selector/1 -> Bus Creator/4  "vx"
  Demux/3 -> Bus Creator/3  "z"
  Selector1/1 -> Bus Creator/5  "vy"
  Bus Creator/1 -> States/1

== system VTOLAutopilotController (minhyun-purdue's conflicted copy 2025-07-07)/Guidance Test Bench/ControlType/Guidance Testbench/Guidance Logic/Subsystem ==
  note: Tilt Angle also determines the state aircraft is in. Thus a unit delay is added
  UAVState : Inport
  Bus Creator : BusCreator  Inputs=6  OutDataTypeStr=Bus: GuidanceStates
  Bus Selector : BusSelector  OutputSignals=Euler,pqr,Ve,Xe,course,RotorParameters.Tilt1
  Gain : Gain
  Unit Delay : UnitDelay  InitialCondition=tiltIni  SampleTime=-1  HasFrameUpgradeWarning=on
  States : Outport
  wires:
  UAVState/1 -> Bus Selector/1
  Bus Selector/1 -> Bus Creator/1  "<Euler>"
  Bus Creator/1 -> States/1
  Bus Selector/3 -> Bus Creator/3  "<Ve>"
  Bus Selector/2 -> Bus Creator/2  "<pqr>"
  Bus Selector/4 -> Bus Creator/4  "<Xe>"
  Bus Selector/5 -> Bus Creator/5  "<course>"
  Gain/1 -> Bus Creator/6  "Tilt"
  Unit Delay/1 -> Gain/1  "Tilt1"
  Bus Selector/6 -> Unit Delay/1  "<Tilt1>"

== system VTOLAutopilotController (minhyun-purdue's conflicted copy 2025-07-07)/Guidance Test Bench/ControlType/Manual Control/Command Interface/Control Rate Transition ==
  FM : Inport
  "ControlMode " : Inport  Port=2
  FixedWingSetpoint : Inport  Port=3
  AACSetpoint : Inport  Port=4
  Position : Inport  Port=5
  Rate Transition{,1..3,5} (5 alike) : RateTransition  OutPortSampleTime=ControlSampleTime
  ctrlMode : Outport
  FixedWingSP : Outport  Port=2
  AACSP : Outport  Port=3
  PositionCmds : Outport  Port=4
  FlightMode : Outport  Port=5
  wires:
  Rate Transition5/1 -> FlightMode/1
  Position/1 -> Rate Transition3/1
  FixedWingSetpoint/1 -> Rate Transition1/1
  Rate Transition3/1 -> PositionCmds/1
  FM/1 -> Rate Transition5/1
  "ControlMode "/1 -> Rate Transition/1
  Rate Transition1/1 -> FixedWingSP/1
  AACSetpoint/1 -> Rate Transition2/1
  Rate Transition2/1 -> AACSP/1
  Rate Transition/1 -> ctrlMode/1

== system VTOLAutopilotController (minhyun-purdue's conflicted copy 2025-07-07)/Guidance Test Bench/ControlType/Manual Control/Command Interface/Subsystem ==
  note: Tilt Angle also determines the state aircraft is in. Thus a unit delay is added
  UAVState : Inport
  Bus Creator : BusCreator  Inputs=6  OutDataTypeStr=Bus: GuidanceStates
  Bus Selector : BusSelector  OutputSignals=Euler,pqr,Ve,Xe,course,RotorParameters.Tilt1
  Gain : Gain
  Unit Delay : UnitDelay  InitialCondition=tiltIni  SampleTime=-1  HasFrameUpgradeWarning=on
  States : Outport
  wires:
  UAVState/1 -> Bus Selector/1
  Bus Selector/1 -> Bus Creator/1  "<Euler>"
  Bus Creator/1 -> States/1
  Bus Selector/3 -> Bus Creator/3  "<Ve>"
  Bus Selector/2 -> Bus Creator/2  "<pqr>"
  Bus Selector/4 -> Bus Creator/4  "<Xe>"
  Bus Selector/5 -> Bus Creator/5  "<course>"
  Bus Selector/6 -> Unit Delay/1  "<Tilt1>"
  Gain/1 -> Bus Creator/6  "Tilt"
  Unit Delay/1 -> Gain/1  "Tilt2"

== system VTOLAutopilotController (minhyun-purdue's conflicted copy 2025-07-07)/Low level controller/Fixed Wing Controller/Fixed Wing Controller Module/Fixed Wing Controller Simulation/AER from Path Manager ==
  In1 : Inport
  Enable : EnablePort
  Out1 : Outport
  wires:
  In1/1 -> Out1/1

== system VTOLAutopilotController (minhyun-purdue's conflicted copy 2025-07-07)/Low level controller/Fixed Wing Controller/Fixed Wing Controller Module/Fixed Wing Controller Simulation/Airspeed-Altitude Controller ==
  note: Airspeed and altitude are controlled independently
      | by ignoring their coupled dynamics.
  Airspeed SP : Inport
  Altitude SP : Inport  Port=2
  Climb Rate SP : Inport  Port=3
  Airspeed : Inport  Port=4
  xyz : Inport  Port=5
  vxyz : Inport  Port=6
  Enable : EnablePort  ShowOutputPort=on
  Airspeed Controller : slpidlib/PID Controller  Controller=PID  Form=Parallel  TimeDomain=Discrete-time  UseExternalTs=off  SampleTime=ControlSampleTime  IntegratorMethod=Trapezoidal  FilterMethod=Forward Euler  ControllerParametersSource=internal  P=FWControlParams.P_AIRSPD  I=FWControlParams.I_AIRSPD+1  UseKiTs=off  D=FWControlParams.D_AIRSPD  UseExternalDerivativeSource=off  N=FWControlParams.N_AIRSPD  UseFilter=on  TunerSelectOption=Transfer Function Based (PID Tuner App)  InitialConditionSource=internal  InitialConditionForIntegrator=0  InitialConditionForFilter=0  DifferentiatorICPrevScaledInput=0  ExternalReset=none  TrackingMode=off  Kt=1  LimitOutput=off  SatLimitsSource=internal  UpperSaturationLimit=Inf  LowerSaturationLimit=0  LinearizeAsGain=on  AntiWindupMode=clamping  Kb=1  LimitIntegrator=off  UpperIntegratorSaturationLimit=inf  LowerIntegratorSaturationLimit=-inf  POutMin=[]  POutMax=[]  IOutMin=[]  IOutMax=[]  DOutMin=[]  DOutMax=[]  NOutMin=[]  NOutMax=[]  SumOutMin=[]  SumOutMax=[]  SaturationOutMin=[]  SaturationOutMax=[]  PParamMin=[]  PParamMax=[]  IParamMin=[]  IParamMax=[]  DParamMin=[]  DParamMax=[]  NParamMin=[]  NParamMax=[]  KbParamMin=[]  KbParamMax=[]  KtParamMin=[]  KtParamMax=[]  KbOutMin=[]  KbOutMax=[]  KtOutMin=[]  KtOutMax=[]  IntegratorOutMin=[]  IntegratorOutMax=[]  FilterOutMin=[]  FilterOutMax=[]  SumI1OutMin=[]  SumI1OutMax=[]  SumI2OutMin=[]  SumI2OutMax=[]  SumI3OutMin=[]  SumI3OutMax=[]  SumI4OutMin=[]  SumI4OutMax=[]  SumDOutMin=[]  SumDOutMax=[]  DifferentiatorOutMin=[]  DifferentiatorOutMax=[]  FilterDiffOutCoefMin=[]  FilterDiffOutCoefMax=[]  ReciprocalOutMin=[]  ReciprocalOutMax=[]  SumDenOutMin=[]  SumDenOutMax=[]  SumNumOutMin=[]  SumNumOutMax=[]  DivideOutMin=[]  DivideOutMax=[]  UdiffTsProdOutMin=[]  UdiffTsProdOutMax=[]  NTsProdOutMin=[]  NTsProdOutMax=[]  UintegralTsProdOutMin=[]  UintegralTsProdOutMax=[]  UngainTsProdOutMin=[]  UngainTsProdOutMax=[]  ClampingZeroOutDataTypeStr=Inherit: Inherit via back propagation  ClampingZeroOutMin=[]  ClampingZeroOutMax=[]  FilterDenConstantOutDataTypeStr=Inherit: Inherit via back propagation  FilterDenConstantOutMin=[]  FilterDenConstantOutMax=[]  PCopyOutDataTypeStr=Inherit: Inherit via back propagation  PCopyOutMin=[]  PCopyOutMax=[]  NCopyOutDataTypeStr=Inherit: Inherit via back propagation  NCopyOutMin=[]  NCopyOutMax=[]  IntegratorContinuousStateAttributes=''  IntegratorStateMustResolveToSignalObject=off  IntegratorRTWStateStorageClass=Auto  FilterContinuousStateAttributes=''  FilterStateMustResolveToSignalObject=off  FilterRTWStateStorageClass=Auto  ParallelPVariant=InternalParameters  IdealPVariant=Disabled  IVariant=InternalParameters  DVariant=InternalParameters  IntegratorVariant=Discrete  SatVariant=Disabled  AWVariant=Passthrough  PCopyVariant=Disabled  TRVariant=Disabled  FdbkBlocksVariant=Forward  IdealPFdbkVariant=Disabled  SatFdbkVariant=Disabled  DerivativeFilterVariant=ForwardEulerFilter  NVariant=InternalParameters  NCopyVariant=Disabled  FilterICVariant=InternalICsFilter  IntegratorICVariant=InternalICs  ExternalResetVariant=Disabled  TRSumVariant=Passthrough  SumFdbkVariant=Disabled  SumVariant=Sum_PID  TsampFilterVariant=InternalTs  TsampNgainVariant=Passthrough  TsampIntegralVariant=Disabled_SignalSpec  ExternalSaturationOutDataTypeStr=Inherit: Same as second input  DerivativeSourceVariant=ErrorSignal  PreIntVariant=InternalPreInt
  Altitude controller : Subsystem
  Climb Rate SP Merge : Merge
  Climb Rate SP from Guidance : Subsystem  TreatAsAtomicUnit=on
  Compare To Constant : simulink/Logic and Bit Operations/Compare To Constant  relop===  const=uint8(1)  OutDataTypeStr=boolean
  Compare To Constant1 : simulink/Logic and Bit Operations/Compare To Constant  relop===  const=uint8(2)  OutDataTypeStr=boolean
  Pitch SP Controller : Subsystem
  Sum1 : Sum  Inputs=|+-
  Pitch SP : Outport
  Throttle : Outport  Port=2
  wires:
  Airspeed SP/1 -> Sum1/1
  Sum1/1 -> Airspeed Controller/1
  Airspeed/1 -> Sum1/2
  Airspeed Controller/1 -> Throttle/1
  Altitude SP/1 -> Altitude controller/1(Alt SP)
  xyz/1 -> Altitude controller/2(xyz)
  vxyz/1 -> Pitch SP Controller/2(vxyz)
  Pitch SP Controller/1(Pitch SP) -> Pitch SP/1
  Enable/1 -> Compare To Constant1/1, Compare To Constant/1
  Compare To Constant/1 -> Altitude controller/Enable
  Compare To Constant1/1 -> Climb Rate SP from Guidance/Enable
  Altitude controller/1(Climb Rate SP) -> Climb Rate SP Merge/1
  Climb Rate SP from Guidance/1(Out1) -> Climb Rate SP Merge/2
  Climb Rate SP Merge/1 -> Pitch SP Controller/1(Climb Rate SP)
  Climb Rate SP/1 -> Climb Rate SP from Guidance/1(Climb Rate SP)
